simulink model "mContinuousTop"  (Simulink 8.0)
settings: Solver=ode45  StartTime=0.0  StopTime=10.0  FixedStep=Auto  RelTol=1e-3
settings Model: FPTRunName=Active  Creator=The MathWorks Inc.  LastModifiedBy=mtocci  ExtModeAutoUpdateStatusClock=off
settings DataIOCC: SignalLoggingSaveFormat=ModelDataLogs  SignalLoggingName=logsOut
settings OptimizationCC: InlineParams=on  InlineInvariantSignals=on  InitFltsAndDblsToZero=on
settings DebuggingCC: SaveWithParameterizedLinksMsg=none  CheckExecutionContextPreStartOutputMsg=on  CheckExecutionContextRuntimeOutputMsg=on  SolverPrmCheckMsg=none  MultiTaskDSMMsg=warning  MultiTaskCondExecSysMsg=none  SigSpecEnsureSampleTimeMsg=none  FcnCallInpInsideContextMsg=Use local settings  StrictBusMsg=ErrorOnBusTreatedAsVector
settings HardwareCC: TargetHWDeviceType=32-bit Generic
settings ModelReferenceCC: UpdateModelReferenceTargets=IfOutOfDate  CheckModelReferenceTargetMessage=none
settings RTWCC: GenerateReport=on  TLCDebug=on  ProcessScript=grt_make_rtw_hook  LaunchReport=on  IncludeERTFirstTime=on
settings CodeAppCC: MaxIdLength=100
settings GRTTargetCC: TargetFcnLib=ansi_tfl_tmw.mat  SharedFunctionMode=Off  CombineOutputUpdateFcns=off

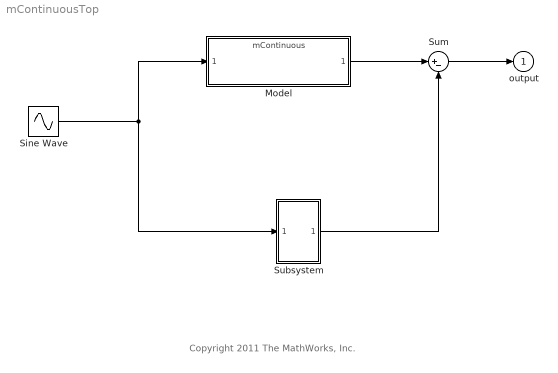
== system mContinuousTop ==
  note: Copyright 2011 The MathWorks, Inc.
  Model : ModelReference  ModelNameDialog=mContinuous  SimulationMode=Accelerator  ModelReferenceVersion=1.85  CopyOfModelName=mContinuous  DefaultDataLogging=on
  Sine Wave : Sin  SampleTime=0
  Subsystem : Subsystem
  Sum : Sum  Inputs=|+-
  output : Outport
  wires:
  Sine Wave/1 -> Model/1, Subsystem/1(In1)
  Subsystem/1(output) -> Sum/2
  Model/1 -> Sum/1
  Sum/1 -> output/1

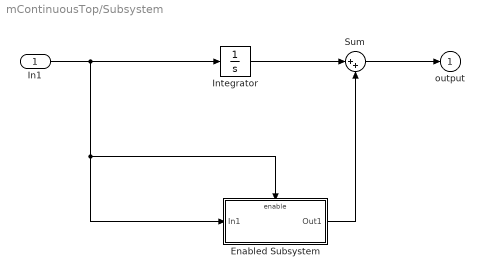
== system mContinuousTop/Subsystem ==
  In1 : Inport
  Enabled Subsystem : Subsystem  TreatAsAtomicUnit=on
  Integrator : Integrator
  Sum : Sum  Inputs=|++
  output : Outport
  wires:
  In1/1 -> Enabled Subsystem/Enable, Enabled Subsystem/1(In1), Integrator/1
  Enabled Subsystem/1(Out1) -> Sum/2
  Sum/1 -> output/1
  Integrator/1 -> Sum/1

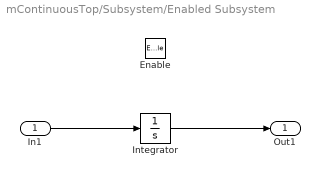
== system mContinuousTop/Subsystem/Enabled Subsystem ==
  In1 : Inport
  Enable : EnablePort  StatesWhenEnabling=reset
  Integrator : Integrator
  Out1 : Outport  InitialOutput=0
  wires:
  Integrator/1 -> Out1/1
  In1/1 -> Integrator/1
